simulink model "UZ_EnDat_be4_adding_bidirectional_clk_shift"  (R2024a)
settings: Solver=FixedStepDiscrete  StartTime=0  StopTime=0.02  FixedStep=1.0E-8  RelTol=1e-3
model workspace (MAT data in the model file):
  Select = 0
libraries: hdlsllib x776, simulink x28, simulink_extras x3
(part 2 of 9)

== system UZ_EnDat_be4_adding_bidirectional_clk_shift/UZ_ENDAT/CRC_Check ==
  set : Inport
  data : Inport  Port=2  OutDataTypeStr=boolean
  clk : Inport  Port=3  OutDataTypeStr=boolean
  Constant : Constant  OutDataTypeStr=boolean  SampleTime=-1
  Constant1 : Constant  Value=0  OutDataTypeStr=boolean  SampleTime=-1
  DFF1 : Subsystem
  DFF2 : Subsystem
  DFF3 : Subsystem
  DFF4 : Subsystem
  DFF5 : Subsystem
  Logical Operator : Logic  Operator=OR  AllPortsSameDT=off  OutDataTypeStr=boolean
  Logical Operator{1..2,5..6} (4 alike) : Logic  AllPortsSameDT=off  OutDataTypeStr=boolean
  Logical Operator3 : Logic  Operator=NOT  AllPortsSameDT=off  OutDataTypeStr=boolean
  Logical Operator4 : Logic  Operator=NOT  AllPortsSameDT=off  OutDataTypeStr=boolean
  Memory : Memory  InheritSampleTime=on
  Memory1 : Memory  InheritSampleTime=on
  Relational Operator : RelationalOperator  Operator===  OutDataTypeStr=boolean  InputSameDT=off
  Relational Operator1 : RelationalOperator  Operator===  OutDataTypeStr=boolean  InputSameDT=off
  Relational Operator2 : RelationalOperator  Operator===  OutDataTypeStr=boolean  InputSameDT=off
  Terminator{,1..3} (4 alike) : Terminator
  crc : Outport
  CRC1 : Outport  Port=2
  CRC2 : Outport  Port=3
  CRC3 : Outport  Port=4
  CRC4 : Outport  Port=5
  CRC5 : Outport  Port=6
  wires:
  Logical Operator/1 -> crc/1
  Logical Operator2/1 -> Logical Operator/2
  Logical Operator1/1 -> Logical Operator/1
  data/1 -> Relational Operator/2, Logical Operator1/1
  Logical Operator3/1 -> Logical Operator1/2
  Logical Operator4/1 -> Logical Operator3/1, Logical Operator2/2
  Logical Operator5/1 -> Memory1/1
  Relational Operator/1 -> DFF1/3(D), Logical Operator6/1
  clk/1 -> DFF1/2(CLK), DFF2/2(CLK), DFF3/2(CLK), DFF5/2(CLK), DFF4/2(CLK)
  set/1 -> Logical Operator6/2, Logical Operator5/2, Logical Operator4/1
  DFF1/1(OQ) -> Relational Operator1/1, CRC1/1
  Logical Operator6/1 -> Memory/1
  Relational Operator1/1 -> DFF2/3(D)
  Relational Operator2/1 -> DFF4/3(D)
  DFF3/1(OQ) -> CRC3/1, Relational Operator2/1
  DFF4/1(OQ) -> DFF5/3(D), CRC4/1
  DFF5/2(NOQ) -> Logical Operator2/1
  DFF5/1(OQ) -> Logical Operator5/1, CRC5/1
  DFF2/1(OQ) -> DFF3/3(D), CRC2/1
  DFF1/2(NOQ) -> Terminator/1
  DFF2/2(NOQ) -> Terminator1/1
  DFF3/2(NOQ) -> Terminator2/1
  DFF4/2(NOQ) -> Terminator3/1
  Constant/1 -> DFF3/1(SET), DFF5/1(SET), DFF4/1(SET), DFF2/1(SET), DFF1/1(SET)
  Constant1/1 -> DFF5/4(RST), DFF4/4(RST), DFF3/4(RST), DFF2/4(RST), DFF1/4(RST)
  Memory/1 -> Relational Operator2/2, Relational Operator1/2
  Memory1/1 -> Relational Operator/1

== system UZ_EnDat_be4_adding_bidirectional_clk_shift/UZ_ENDAT/DATA2CLOCKSYNCER ==
  In1 : Inport
  FAKTOR : Inport  Port=2
  Constant : Constant  Value=100  OutDataTypeStr=uint16  SampleTime=-1
  Constant1 : Constant  Value=45  OutDataTypeStr=uint16  SampleTime=-1
  Constant2 : Constant  Value=2  OutDataTypeStr=uint16  SampleTime=-1
  Constant23 : Constant  Value=20  OutDataTypeStr=uint16  SampleTime=-1
  Constant24 : Constant  Value=29  OutDataTypeStr=uint16  SampleTime=-1
  Constant3 : Constant  Value=12  OutDataTypeStr=uint16  SampleTime=-1
  Constant4 : Constant  Value=4  OutDataTypeStr=uint16  SampleTime=-1
  Constant7 : Constant  Value=8  OutDataTypeStr=uint16  SampleTime=-1
  Display15 : Display
  Divide : Product  Inputs=*/  OutDataTypeStr=uint16  RndMeth=Simplest  SaturateOnIntegerOverflow=on
  Multiport Switch1 : MultiPortSwitch  DataPortOrder=Zero-based contiguous  Inputs=7  DataPortIndices={8,16,32,64}  zeroidx=on  SaturateOnIntegerOverflow=off  InputSameDT=off
  Product : Product  RndMeth=Simplest  SaturateOnIntegerOverflow=on  OutDataTypeStr=Inherit: Same as first input
  Out1 : Outport
  wires:
  In1/1 -> Multiport Switch1/1
  FAKTOR/1 -> Product/2
  Constant/1 -> Divide/2
  Multiport Switch1/1 -> Product/1
  Product/1 -> Divide/1
  Constant2/1 -> Multiport Switch1/2
  Constant4/1 -> Multiport Switch1/3
  Constant7/1 -> Multiport Switch1/4
  Constant3/1 -> Multiport Switch1/5
  Constant23/1 -> Multiport Switch1/6
  Constant24/1 -> Multiport Switch1/7
  Constant1/1 -> Multiport Switch1/8
  Divide/1 -> Display15/1, Out1/1

== system UZ_EnDat_be4_adding_bidirectional_clk_shift/UZ_ENDAT/DATAFLOWCHGER ==
  CLKSEL : Inport
  FACTOR : Inport  Port=2
  Constant : Constant  Value=100  OutDataTypeStr=uint16  SampleTime=-1
  Constant{14..18,27..28} (7 alike) : Constant  Value=10  OutDataTypeStr=uint16  SampleTime=-1
  Divide : Product  Inputs=*/  InputSameDT=on  OutDataTypeStr=uint16  RndMeth=Simplest  SaturateOnIntegerOverflow=on
  Multiport Switch2 : MultiPortSwitch  DataPortOrder=Zero-based contiguous  Inputs=7  DataPortIndices={8,16,32,64}  zeroidx=on  SaturateOnIntegerOverflow=off  InputSameDT=off
  Product : Product  RndMeth=Simplest  SaturateOnIntegerOverflow=on  OutDataTypeStr=Inherit: Same as first input
  Output : Outport
  wires:
  Product/1 -> Divide/1
  CLKSEL/1 -> Multiport Switch2/1
  FACTOR/1 -> Product/2
  Constant/1 -> Divide/2
  Divide/1 -> Output/1
  Multiport Switch2/1 -> Product/1
  Constant15/1 -> Multiport Switch2/2
  Constant16/1 -> Multiport Switch2/3
  Constant17/1 -> Multiport Switch2/4
  Constant18/1 -> Multiport Switch2/5
  Constant27/1 -> Multiport Switch2/6
  Constant28/1 -> Multiport Switch2/7
  Constant14/1 -> Multiport Switch2/8

== system UZ_EnDat_be4_adding_bidirectional_clk_shift/UZ_ENDAT/DIFFBUILDER ==
  DATAT0 : Inport
  DATAT1 : Inport  Port=2
  DATAT2 : Inport  Port=3
  Trigger : TriggerPort  VariantControl=(inherit)  OutputDataType=int8  InitialTriggerSignalState=positive
  Subtract : Sum  Inputs=+-  OutDataTypeStr=int32  InputSameDT=on  RndMeth=Simplest
  Subtract1 : Sum  Inputs=+-  OutDataTypeStr=int32  InputSameDT=on  RndMeth=Simplest
  DIFT1T0 : Outport  InitialOutput=0
  DIFT2T0 : Outport  Port=2  InitialOutput=0
  wires:
  DATAT1/1 -> Subtract/2
  DATAT0/1 -> Subtract/1, Subtract1/1
  Subtract/1 -> DIFT1T0/1
  Subtract1/1 -> DIFT2T0/1
  DATAT2/1 -> Subtract1/2

== system UZ_EnDat_be4_adding_bidirectional_clk_shift/UZ_ENDAT/INITIALOFF ==
  CLKAUX : Inport
  CLK : Inport  Port=2
  DATAWR : Inport  Port=3
  DATA : Inport  Port=4
  CLKWR : Inport  Port=5
  FACTOR : Inport  Port=6
  Constant : Constant  Value=0  OutDataTypeStr=boolean  SampleTime=-1
  Display : Display
  Memory : Memory  InheritSampleTime=on
  Multiport Switch{,1..3} (4 alike) : MultiPortSwitch  DataPortOrder=Zero-based contiguous  Inputs=2  zeroidx=on  SaturateOnIntegerOverflow=off  InputSameDT=off
  Relational Operator : RelationalOperator  Operator=<  OutDataTypeStr=boolean  InputSameDT=off
  Subsystem : Subsystem
  Subsystem6 : Subsystem
  CLK_OUT : Outport
  DATAWR_OUT : Outport  Port=2
  DATA_OUT : Outport  Port=3
  CLKWR_OUT : Outport  Port=4
  wires:
  Relational Operator/1 -> Multiport Switch3/1, Multiport Switch2/1, Multiport Switch1/1, Multiport Switch/1, Memory/1
  CLK/1 -> Multiport Switch/2
  Multiport Switch/1 -> CLK_OUT/1
  CLKAUX/1 -> Subsystem/Trigger
  Constant/1 -> Multiport Switch3/3, Multiport Switch2/3, Multiport Switch1/3, Multiport Switch/3
  Multiport Switch1/1 -> DATAWR_OUT/1
  Multiport Switch2/1 -> DATA_OUT/1
  Multiport Switch3/1 -> CLKWR_OUT/1
  DATAWR/1 -> Multiport Switch1/2
  DATA/1 -> Multiport Switch2/2
  CLKWR/1 -> Multiport Switch3/2
  Subsystem6/1(out) -> Relational Operator/2
  FACTOR/1 -> Subsystem6/1(FACTOR)
  Subsystem/1(count) -> Display/1, Relational Operator/1
  Memory/1 -> Subsystem/1(In1)

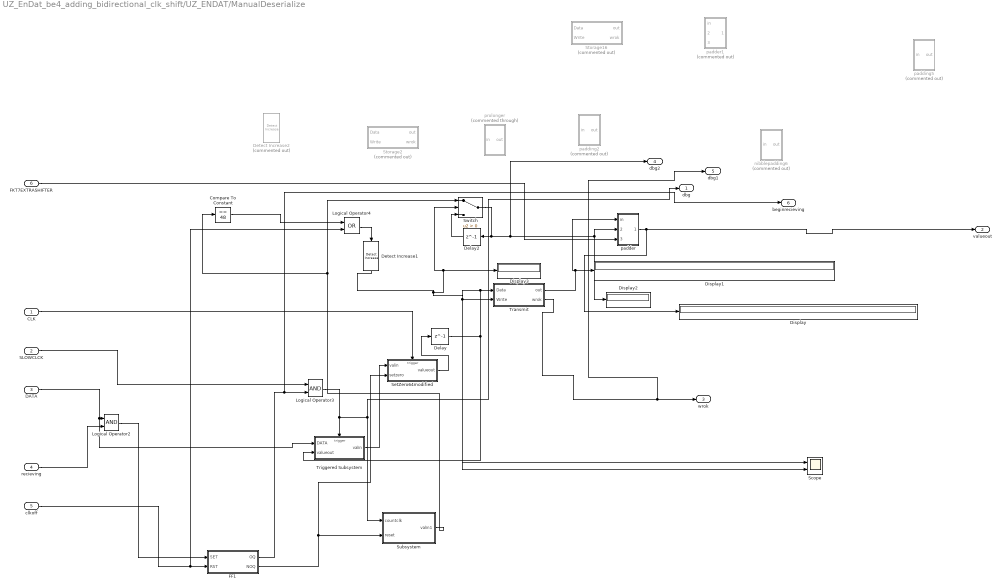
== system UZ_EnDat_be4_adding_bidirectional_clk_shift/UZ_ENDAT/ManualDeserialize ==
  CLK : Inport
  SLOWCLCK : Inport  Port=2
  DATA : Inport  Port=3
  recieving : Inport  Port=4  OutMin=0  OutMax=1  OutDataTypeStr=boolean
  clkoff : Inport  Port=5  OutMin=0  OutMax=1  OutDataTypeStr=boolean
  FKT7EXTRASHIFTER : Inport  Port=6
  Compare To Constant : hdlsllib/Logic and Bit Operations/Compare To Constant  relop===  const=48  OutDataTypeStr=boolean
  Delay : Delay  DelayLength=1
  Delay2 : Delay  DelayLength=1
  Detect Increase1 : simulink/Logic and Bit Operations/Detect Increase  vinit=0  OutDataTypeStr=boolean
      settings: LibrarySourceBlock=|
      | hdlsllib/Logic and Bit
      | Operations/Detect
      | Increase
  Detect Increase2 : simulink/Logic and Bit Operations/Detect Increase  Commented=on  vinit=0.0  InputProcessing=Columns as channels (frame based)  OutDataTypeStr=boolean
      settings: LibrarySourceBlock=|
      | hdlsllib/Logic and Bit
      | Operations/Detect
      | Increase
  Display{,1..3} (4 alike) : Display
      Display settings: Format=binary (Stored Integer)
      Display1 settings: Format=binary (Stored Integer)
  FF1 : Subsystem  TreatAsAtomicUnit=on
      settings: LibrarySourceBlock=|
      | hdlsllib/Ports &
      | Subsystems/Triggered
      | Subsystem
  Logical Operator2 : Logic  AllPortsSameDT=off  OutDataTypeStr=boolean
  Logical Operator3 : Logic  AllPortsSameDT=off  OutDataTypeStr=boolean
  Logical Operator4 : Logic  Operator=OR  AllPortsSameDT=off  OutDataTypeStr=boolean
  Scope : Scope  NumInputPorts=2
  SetZero64modified : Subsystem
  Storage16 : Subsystem  Commented=on
      settings: LibrarySourceBlock=|
      | hdlsllib/Ports &
      | Subsystems/Subsystem
  Storage2 : Subsystem  Commented=on
      settings: LibrarySourceBlock=|
      | hdlsllib/Ports &
      | Subsystems/Subsystem
  Subsystem : Subsystem
  Switch : Switch  Criteria=u2 > Threshold  SaturateOnIntegerOverflow=off  InputSameDT=off
  Transmit : Subsystem
      settings: LibrarySourceBlock=|
      | hdlsllib/Ports &
      | Subsystems/Subsystem
  Triggered Subsystem : Subsystem  TreatAsAtomicUnit=on
      settings: LibrarySourceBlock=|
      | hdlsllib/Ports &
      | Subsystems/Triggered
      | Subsystem
  nibblepadding6 : Subsystem  Commented=on
  padder : Subsystem
  padder1 : Subsystem  Commented=on
  padding2 : Subsystem  Commented=on
  padding5 : Subsystem  Commented=on
  prolonger : Subsystem  Commented=through
  dbg : Outport  OutDataTypeStr=boolean  VectorParamsAs1DForOutWhenUnconnected=off
  valueout : Outport  Port=2  OutDataTypeStr=uint64
  wrok : Outport  Port=3  OutDataTypeStr=boolean
  dbg2 : Outport  Port=4  OutDataTypeStr=uint8  VectorParamsAs1DForOutWhenUnconnected=off
  dbg1 : Outport  Port=5  OutDataTypeStr=boolean  VectorParamsAs1DForOutWhenUnconnected=off
  beginrecieving : Outport  Port=6  OutDataTypeStr=boolean  VectorParamsAs1DForOutWhenUnconnected=off
  wires:
  SetZero64modified/1(valueout) -> Delay/1
  CLK/1 -> SetZero64modified/Trigger
  SLOWCLCK/1 -> Logical Operator3/1
  Triggered Subsystem/1(valin) -> SetZero64modified/1(valin)
  Logical Operator3/1 -> dbg/1, Subsystem/1(countclk), Triggered Subsystem/Trigger
  Logical Operator2/1 -> FF1/1(SET)
  FF1/1(OQ) -> beginrecieving/1, Logical Operator3/2
  recieving/1 -> Logical Operator2/2
  FF1/2(NOQ) -> Subsystem/2(reset), SetZero64modified/2(setzero)
  Compare To Constant/1 -> Logical Operator4/1
  Delay2/1 -> Switch/3
  clkoff/1 -> Logical Operator4/2, FF1/2(RST)
  DATA/1 -> Triggered Subsystem/1(DATA), Logical Operator2/1
  Delay/1 -> Transmit/1(Data), Scope/2, Triggered Subsystem/2(valueout)
  Transmit/1(out) -> padder/1(in), Display1/1
  padder/1(out) -> valueout/1, Display/1
  Switch/1 -> Delay2/1, dbg2/1, padder/2(CTR), Display2/1
  Transmit/2(wrok) -> dbg1/1, wrok/1
  FKT7EXTRASHIFTER/1 -> padder/3(in1)
  Logical Operator4/1 -> Detect Increase1/1
  Subsystem/1(valin1) -> Switch/1, Compare To Constant/1
  Detect Increase1/1 -> Transmit/2(Write), Scope/1, Switch/2, Display3/1

== system UZ_EnDat_be4_adding_bidirectional_clk_shift/UZ_ENDAT/ManualSerializeWrap ==
  CLK : Inport
  SLOWCLCK : Inport  Port=2
  DATA : Inport  Port=3
  reset : Inport  Port=4
  Enable : EnablePort
  ManualSerializer : Subsystem
      settings: LibrarySourceBlock=|
      | hdlsllib/Ports &
      | Subsystems/Subsystem
  valin : Outport  InitialOutput=0
  wires:
  CLK/1 -> ManualSerializer/1(CLK)
  DATA/1 -> ManualSerializer/3(DATA)
  reset/1 -> ManualSerializer/4(reset)
  SLOWCLCK/1 -> ManualSerializer/2(SLOWCLCK)
  ManualSerializer/1(valin) -> valin/1

== system UZ_EnDat_be4_adding_bidirectional_clk_shift/UZ_ENDAT/OUTPUTCONTROLCONTINIOUS ==
  CLKCNT : Inport
  CLKS2DATAFLOWCHG : Inport  Port=2
  CLK2ENDOFTRANSMISSION : Inport  Port=3
  OPENCOM : Inport  Port=4
  CLKCNTNOSTOP : Inport  Port=5
  RECOVERYTIME : Inport  Port=6  OutDataTypeStr=uint16
  Add : Sum  OutDataTypeStr=uint16  AccumDataTypeStr=uint16
  Constant : Constant  Value=0  OutDataTypeStr=uint8  SampleTime=-1
  Logical Operator : Logic  Operator=OR  AllPortsSameDT=off  OutDataTypeStr=boolean
  Logical Operator1 : Logic  AllPortsSameDT=off  OutDataTypeStr=boolean
  Logical Operator6 : Logic  Operator=NOT  Inputs=3  AllPortsSameDT=off  OutDataTypeStr=boolean
  Relational Operator : RelationalOperator  Operator=<=  OutDataTypeStr=boolean  RndMeth=Simplest  InputSameDT=off
  Relational Operator1 : RelationalOperator  OutDataTypeStr=boolean  RndMeth=Simplest  InputSameDT=off
  Relational Operator2 : RelationalOperator  OutDataTypeStr=boolean  RndMeth=Simplest  InputSameDT=off
  Relational Operator3 : RelationalOperator  OutDataTypeStr=boolean  RndMeth=Simplest  InputSameDT=off
  CLKOFF : Outport  OutDataTypeStr=boolean
  DATAINV : Outport  Port=2  OutDataTypeStr=boolean
  RESETCNT : Outport  Port=3  OutDataTypeStr=boolean
  wires:
  CLKCNT/1 -> Relational Operator1/1, Relational Operator2/1, Relational Operator/1
  CLKS2DATAFLOWCHG/1 -> Relational Operator/2
  Relational Operator/1 -> Logical Operator1/1
  CLK2ENDOFTRANSMISSION/1 -> Add/1, Relational Operator1/2
  Relational Operator1/1 -> Logical Operator/2
  Logical Operator/1 -> CLKOFF/1
  OPENCOM/1 -> Logical Operator6/1
  Logical Operator6/1 -> Logical Operator/1
  Relational Operator2/1 -> Logical Operator1/2
  Constant/1 -> Relational Operator2/2
  Logical Operator1/1 -> DATAINV/1
  RECOVERYTIME/1 -> Add/2
  Add/1 -> Relational Operator3/2
  Relational Operator3/1 -> RESETCNT/1
  CLKCNTNOSTOP/1 -> Relational Operator3/1

== system UZ_EnDat_be4_adding_bidirectional_clk_shift/UZ_ENDAT/RECOVERYTIMESELECTOR ==
  note: 200khz = 6
      | 1,5mhz = 12
      | 3 mhz = 8
  In1 : Inport
  FAKTOR : Inport  Port=2
  Constant : Constant  Value=100  OutDataTypeStr=uint16  SampleTime=-1
  Constant19 : Constant  Value=96  OutDataTypeStr=uint16  SampleTime=-1
  Constant20 : Constant  Value=48  OutDataTypeStr=uint16  SampleTime=-1
  Constant21 : Constant  Value=192  OutDataTypeStr=uint16  SampleTime=-1
  Constant22 : Constant  Value=255  OutDataTypeStr=uint16  SampleTime=-1
  Constant25 : Constant  Value=24  OutDataTypeStr=uint16  SampleTime=-1
  Constant26 : Constant  Value=12  OutDataTypeStr=uint16  SampleTime=-1
  Constant5 : Constant  Value=6  OutDataTypeStr=uint16  SampleTime=-1
  Divide : Product  Inputs=*/  InputSameDT=on  OutDataTypeStr=uint16  RndMeth=Simplest  SaturateOnIntegerOverflow=on
  Multiport Switch3 : MultiPortSwitch  DataPortOrder=Zero-based contiguous  Inputs=7  DataPortIndices={8,16,32,64}  zeroidx=on  SaturateOnIntegerOverflow=off  InputSameDT=off
  Product : Product  RndMeth=Simplest  SaturateOnIntegerOverflow=on  OutDataTypeStr=Inherit: Same as first input
  Out1 : Outport
  wires:
  In1/1 -> Multiport Switch3/1
  Constant5/1 -> Multiport Switch3/8
  FAKTOR/1 -> Product/2
  Constant/1 -> Divide/2
  Divide/1 -> Out1/1
  Multiport Switch3/1 -> Product/1
  Product/1 -> Divide/1
  Constant26/1 -> Multiport Switch3/7
  Constant25/1 -> Multiport Switch3/6
  Constant20/1 -> Multiport Switch3/5
  Constant19/1 -> Multiport Switch3/4
  Constant21/1 -> Multiport Switch3/3
  Constant22/1 -> Multiport Switch3/2

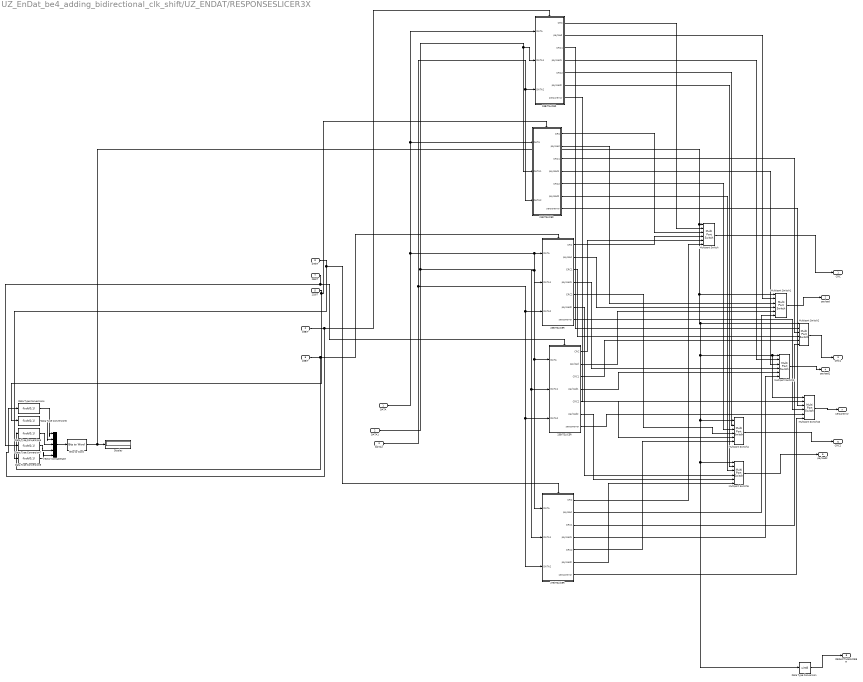
== system UZ_EnDat_be4_adding_bidirectional_clk_shift/UZ_ENDAT/RESPONSESLICER3X ==
  DATA : Inport
  DATA1 : Inport  Port=2
  DATA2 : Inport  Port=3
  19BIT : Inport  Port=4  OutDataTypeStr=boolean
  21BIT : Inport  Port=5  OutDataTypeStr=boolean
  23BIT : Inport  Port=6  OutDataTypeStr=boolean
  25BIT : Inport  Port=7  OutDataTypeStr=boolean
  27BIT : Inport  Port=8  OutDataTypeStr=boolean
  19BITSLICER : Subsystem
  21BITSLICER : Subsystem
  23BITSLICER : Subsystem
  25BITSLICER : Subsystem
  27BITSLICER : Subsystem
  Bits to Word : hdlsllib/Logic and Bit Operations/Bits to Word
  Data Type Conversion : DataTypeConversion  OutDataTypeStr=uint8  RndMeth=Nearest  SaturateOnIntegerOverflow=off
  Data Type Conversion{4..8} (5 alike) : DataTypeConversion  OutMax=1  OutDataTypeStr=fixdt(0,1)  SaturateOnIntegerOverflow=off  RndMeth=Floor
  Display : Display
  Multiport Switch{,1..5,10} (7 alike) : MultiPortSwitch  DataPortOrder=Specify indices  Inputs=5  DataPortIndices={1,2,4,8,16}  DiagnosticForDefault=Warning  RndMeth=Simplest  SaturateOnIntegerOverflow=off  InputSameDT=off
  Vector Concatenate : Concatenate  NumInputs=5
  CRC : Outport
  payload : Outport  Port=2
  CRC1 : Outport  Port=3
  payload1 : Outport  Port=4
  CRC2 : Outport  Port=5
  payload2 : Outport  Port=6
  sensorerror : Outport  Port=7  OutDataTypeStr=boolean
  DBGACTIVENUMBER : Outport  Port=8
  wires:
  23BITSLICER/1(CRC) -> Multiport Switch/4
  DATA1/1 -> 19BITSLICER/2(DATA1), 21BITSLICER/2(DATA1), 23BITSLICER/2(DATA1), 27BITSLICER/2(DATA1), 25BITSLICER/2(DATA1)
  DATA2/1 -> 21BITSLICER/3(DATA2), 19BITSLICER/3(DATA2), 23BITSLICER/3(DATA2), 27BITSLICER/3(DATA2), 25BITSLICER/3(DATA2)
  DATA/1 -> 19BITSLICER/1(DATA), 21BITSLICER/1(DATA), 23BITSLICER/1(DATA), 27BITSLICER/1(DATA), 25BITSLICER/1(DATA)
  Multiport Switch2/1 -> CRC1/1
  Multiport Switch3/1 -> payload1/1
  Multiport Switch4/1 -> CRC2/1
  Multiport Switch5/1 -> payload2/1
  Multiport Switch1/1 -> payload/1
  Multiport Switch/1 -> CRC/1
  19BIT/1 -> 19BITSLICER/Enable, Data Type Conversion4/1
  Data Type Conversion6/1 -> Vector Concatenate/3
  25BIT/1 -> Data Type Conversion7/1, 25BITSLICER/Enable
  Vector Concatenate/1 -> Bits to Word/1
  23BIT/1 -> 23BITSLICER/Enable, Data Type Conversion6/1
  Data Type Conversion4/1 -> Vector Concatenate/1
  Data Type Conversion7/1 -> Vector Concatenate/4
  27BIT/1 -> 27BITSLICER/Enable, Data Type Conversion8/1
  Data Type Conversion5/1 -> Vector Concatenate/2
  21BIT/1 -> 21BITSLICER/Enable, Data Type Conversion5/1
  Data Type Conversion8/1 -> Vector Concatenate/5
  19BITSLICER/1(CRC) -> Multiport Switch/2
  21BITSLICER/1(CRC) -> Multiport Switch/3
  25BITSLICER/1(CRC) -> Multiport Switch/5
  27BITSLICER/1(CRC) -> Multiport Switch/6
  23BITSLICER/2(payload) -> Multiport Switch1/4
  19BITSLICER/2(payload) -> Multiport Switch1/2
  21BITSLICER/2(payload) -> Multiport Switch1/3
  25BITSLICER/2(payload) -> Multiport Switch1/5
  27BITSLICER/2(payload) -> Multiport Switch1/6
  23BITSLICER/3(CRC1) -> Multiport Switch2/4
  21BITSLICER/3(CRC1) -> Multiport Switch2/3
  19BITSLICER/3(CRC1) -> Multiport Switch2/2
  25BITSLICER/3(CRC1) -> Multiport Switch2/5
  27BITSLICER/3(CRC1) -> Multiport Switch2/6
  23BITSLICER/4(payload1) -> Multiport Switch3/4
  21BITSLICER/4(payload1) -> Multiport Switch3/3
  19BITSLICER/4(payload1) -> Multiport Switch3/2
  25BITSLICER/4(payload1) -> Multiport Switch3/5
  27BITSLICER/4(payload1) -> Multiport Switch3/6
  23BITSLICER/5(CRC2) -> Multiport Switch4/4
  19BITSLICER/5(CRC2) -> Multiport Switch4/2
  21BITSLICER/5(CRC2) -> Multiport Switch4/3
  25BITSLICER/5(CRC2) -> Multiport Switch4/5
  27BITSLICER/5(CRC2) -> Multiport Switch4/6
  23BITSLICER/6(payload2) -> Multiport Switch5/4
  19BITSLICER/6(payload2) -> Multiport Switch5/2
  21BITSLICER/6(payload2) -> Multiport Switch5/3
  25BITSLICER/6(payload2) -> Multiport Switch5/5
  27BITSLICER/6(payload2) -> Multiport Switch5/6
  Multiport Switch10/1 -> sensorerror/1
  25BITSLICER/7(sensorerror) -> Multiport Switch10/5
  27BITSLICER/7(sensorerror) -> Multiport Switch10/6
  23BITSLICER/7(sensorerror) -> Multiport Switch10/4
  21BITSLICER/7(sensorerror) -> Multiport Switch10/3
  19BITSLICER/7(sensorerror) -> Multiport Switch10/2
  Data Type Conversion/1 -> DBGACTIVENUMBER/1
  Bits to Word/1 -> Data Type Conversion/1, Multiport Switch5/1, Multiport Switch4/1, Multiport Switch10/1, Multiport Switch3/1, Multiport Switch2/1, Multiport Switch1/1, Multiport Switch/1, Display/1

== system UZ_EnDat_be4_adding_bidirectional_clk_shift/UZ_ENDAT/SetZeroBool ==
  valin : Inport
  setzero : Inport  Port=2  OutDataTypeStr=boolean
  Trigger : TriggerPort  TriggerType=either  VariantControl=(inherit)
  Constant1 : Constant  OutDataTypeStr=boolean  SampleTime=-1
  Constant2 : Constant  Value=0  OutDataTypeStr=boolean  SampleTime=-1
  Index Vector1 : MultiPortSwitch  DataPortOrder=Zero-based contiguous  Inputs=2  zeroidx=on  SaturateOnIntegerOverflow=off  InputSameDT=off
  Logical Operator : Logic  AllPortsSameDT=off  OutDataTypeStr=boolean
  valueout : Outport  InitialOutput=1  VectorParamsAs1DForOutWhenUnconnected=off
  wires:
  Index Vector1/1 -> Logical Operator/1
  valin/1 -> Logical Operator/2
  Logical Operator/1 -> valueout/1
  Constant1/1 -> Index Vector1/2
  Constant2/1 -> Index Vector1/3
  setzero/1 -> Index Vector1/1

== system UZ_EnDat_be4_adding_bidirectional_clk_shift/UZ_ENDAT/SetZeroBool1 ==
  valin : Inport
  setzero : Inport  Port=2  OutDataTypeStr=boolean
  Trigger : TriggerPort  TriggerType=either  VariantControl=(inherit)
  Constant1 : Constant  OutDataTypeStr=boolean  SampleTime=-1
  Constant2 : Constant  Value=0  OutDataTypeStr=boolean  SampleTime=-1
  Index Vector1 : MultiPortSwitch  DataPortOrder=Zero-based contiguous  Inputs=2  zeroidx=on  SaturateOnIntegerOverflow=off  InputSameDT=off
  Logical Operator : Logic  AllPortsSameDT=off  OutDataTypeStr=boolean
  valueout : Outport  InitialOutput=1  VectorParamsAs1DForOutWhenUnconnected=off
  wires:
  Index Vector1/1 -> Logical Operator/1
  valin/1 -> Logical Operator/2
  Logical Operator/1 -> valueout/1
  Constant1/1 -> Index Vector1/2
  Constant2/1 -> Index Vector1/3
  setzero/1 -> Index Vector1/1

== system UZ_EnDat_be4_adding_bidirectional_clk_shift/UZ_ENDAT/SetZeroBool2 ==
  valin : Inport
  setzero : Inport  Port=2  OutDataTypeStr=boolean
  Trigger : TriggerPort  TriggerType=either  VariantControl=(inherit)
  Constant1 : Constant  OutDataTypeStr=boolean  SampleTime=-1
  Constant2 : Constant  Value=0  OutDataTypeStr=boolean  SampleTime=-1
  Index Vector1 : MultiPortSwitch  DataPortOrder=Zero-based contiguous  Inputs=2  zeroidx=on  SaturateOnIntegerOverflow=off  InputSameDT=off
  Logical Operator : Logic  AllPortsSameDT=off  OutDataTypeStr=boolean
  valueout : Outport  InitialOutput=1  VectorParamsAs1DForOutWhenUnconnected=off
  wires:
  Index Vector1/1 -> Logical Operator/1
  valin/1 -> Logical Operator/2
  Logical Operator/1 -> valueout/1
  Constant1/1 -> Index Vector1/2
  Constant2/1 -> Index Vector1/3
  setzero/1 -> Index Vector1/1

== system UZ_EnDat_be4_adding_bidirectional_clk_shift/UZ_ENDAT/SetZeroBool3 ==
  valin : Inport
  setzero : Inport  Port=2  OutDataTypeStr=boolean
  Trigger : TriggerPort  TriggerType=either  VariantControl=(inherit)
  Constant1 : Constant  OutDataTypeStr=boolean  SampleTime=-1
  Constant2 : Constant  Value=0  OutDataTypeStr=boolean  SampleTime=-1
  Index Vector1 : MultiPortSwitch  DataPortOrder=Zero-based contiguous  Inputs=2  zeroidx=on  SaturateOnIntegerOverflow=off  InputSameDT=off
  Logical Operator : Logic  AllPortsSameDT=off  OutDataTypeStr=boolean
  valueout : Outport  InitialOutput=1  VectorParamsAs1DForOutWhenUnconnected=off
  wires:
  Index Vector1/1 -> Logical Operator/1
  valin/1 -> Logical Operator/2
  Logical Operator/1 -> valueout/1
  Constant1/1 -> Index Vector1/2
  Constant2/1 -> Index Vector1/3
  setzero/1 -> Index Vector1/1

== system UZ_EnDat_be4_adding_bidirectional_clk_shift/UZ_ENDAT/SetZeroBool4 ==
  valin : Inport
  setzero : Inport  Port=2  OutDataTypeStr=boolean
  Trigger : TriggerPort  TriggerType=either  VariantControl=(inherit)
  Constant1 : Constant  OutDataTypeStr=boolean  SampleTime=-1
  Constant2 : Constant  Value=0  OutDataTypeStr=boolean  SampleTime=-1
  Index Vector1 : MultiPortSwitch  DataPortOrder=Zero-based contiguous  Inputs=2  zeroidx=on  SaturateOnIntegerOverflow=off  InputSameDT=off
  Logical Operator : Logic  AllPortsSameDT=off  OutDataTypeStr=boolean
  valueout : Outport  InitialOutput=1  VectorParamsAs1DForOutWhenUnconnected=off
  wires:
  Index Vector1/1 -> Logical Operator/1
  valin/1 -> Logical Operator/2
  Logical Operator/1 -> valueout/1
  Constant1/1 -> Index Vector1/2
  Constant2/1 -> Index Vector1/3
  setzero/1 -> Index Vector1/1

== system UZ_EnDat_be4_adding_bidirectional_clk_shift/UZ_ENDAT/SetZeroBool5 ==
  valin : Inport
  setzero : Inport  Port=2  OutDataTypeStr=boolean
  Trigger : TriggerPort  TriggerType=either  VariantControl=(inherit)
  Constant1 : Constant  OutDataTypeStr=boolean  SampleTime=-1
  Constant2 : Constant  Value=0  OutDataTypeStr=boolean  SampleTime=-1
  Index Vector1 : MultiPortSwitch  DataPortOrder=Zero-based contiguous  Inputs=2  zeroidx=on  SaturateOnIntegerOverflow=off  InputSameDT=off
  Logical Operator : Logic  AllPortsSameDT=off  OutDataTypeStr=boolean
  valueout : Outport  InitialOutput=1  VectorParamsAs1DForOutWhenUnconnected=off
  wires:
  Index Vector1/1 -> Logical Operator/1
  valin/1 -> Logical Operator/2
  Logical Operator/1 -> valueout/1
  Constant1/1 -> Index Vector1/2
  Constant2/1 -> Index Vector1/3
  setzero/1 -> Index Vector1/1

== system UZ_EnDat_be4_adding_bidirectional_clk_shift/UZ_ENDAT/Storage16 ==
  Data : Inport
  Write : Inport  Port=2  OutDataTypeStr=boolean
  Compare To Zero : hdlsllib/Logic and Bit Operations/Compare To Zero  relop===  OutDataTypeStr=boolean
  Logical Operator : Logic  Operator=NOT  AllPortsSameDT=off  OutDataTypeStr=boolean
  Logical Operator1 : Logic  Inputs=3  AllPortsSameDT=off  OutDataTypeStr=boolean
  Logical Operator2 : Logic  Operator=NOT  AllPortsSameDT=off  OutDataTypeStr=boolean
  Logical Operator3 : Logic  AllPortsSameDT=off  OutDataTypeStr=boolean
  Relational Operator : RelationalOperator  Operator===  OutDataTypeStr=boolean  InputSameDT=off
  Single Port RAM System : hdlsllib/HDL RAMs/Single Port RAM System  RAMType=Single port  AsyncRead=off  WriteOutputValue=Old data  RAMInitialValue=0  allowBusInputs=off  WritesHaveOutput=on  NumReads=0  NumWrites=1  SimulateUsing=Code generation
  adress : Constant  Value=5  OutDataTypeStr=uint8  SampleTime=-1
  out : Outport
  wrok : Outport  Port=2  OutDataTypeStr=boolean
  wires:
  Single Port RAM System/1 -> Relational Operator/1, out/1
  Data/1 -> Compare To Zero/1, Single Port RAM System/1, Relational Operator/2
  adress/1 -> Single Port RAM System/2
  Relational Operator/1 -> Logical Operator3/1, Logical Operator/1
  Logical Operator/1 -> Logical Operator1/2
  Write/1 -> Logical Operator1/1
  Compare To Zero/1 -> Logical Operator2/1
  Logical Operator2/1 -> Logical Operator3/2, Logical Operator1/3
  Logical Operator1/1 -> Single Port RAM System/3
  Logical Operator3/1 -> wrok/1

== system UZ_EnDat_be4_adding_bidirectional_clk_shift/UZ_ENDAT/Subsystem1 ==
  in : Inport
  Enable : EnablePort
  Bits to Word1 : hdlsllib/Logic and Bit Operations/Bits to Word
  out : Outport  InitialOutput=0
  wires:
  Bits to Word1/1 -> out/1
  in/1 -> Bits to Word1/1

== system UZ_EnDat_be4_adding_bidirectional_clk_shift/UZ_ENDAT/Subsystem6 ==
  In1 : Inport  OutDataTypeStr=uint16
  FACTOR : Inport  Port=2  OutMin=0  OutMax=60000
  Constant : Constant  Value=100  OutDataTypeStr=uint16  SampleTime=-1
  Divide : Product  Inputs=*/  OutDataTypeStr=uint16  RndMeth=Simplest  SaturateOnIntegerOverflow=on
  Product : Product  OutDataTypeStr=uint16  RndMeth=Simplest  SaturateOnIntegerOverflow=on
  Out1 : Outport
  wires:
  In1/1 -> Product/1
  FACTOR/1 -> Product/2
  Constant/1 -> Divide/2
  Product/1 -> Divide/1
  Divide/1 -> Out1/1

== system UZ_EnDat_be4_adding_bidirectional_clk_shift/UZ_ENDAT/ageprovider ==
  wrok : Inport  OutDataTypeStr=boolean
  recieving : Inport  Port=2  OutDataTypeStr=boolean
  altmode : Inport  Port=3  OutDataTypeStr=boolean
  Constant : Constant  Value=10  OutDataTypeStr=uint8  SampleTime=-1
  Detect Increase1 : simulink/Logic and Bit Operations/Detect Increase  vinit=0  OutDataTypeStr=boolean
      settings: LibrarySourceBlock=|
      | hdlsllib/Logic and Bit
      | Operations/Detect
      | Increase
  Display : Display
  HDL Counter : hdlsllib/Sources/HDL Counter  CountType=Count limited  CountInit=0  CountStep=1  CountMax=65535  CountFromType=Initial value  CountFrom=0  CountResetPort=on  CountLoadPort=off  CountEnbPort=on  CountDirPort=off  CountHitOutputPort=off  CountDataType=Unsigned  CountWordLen=16  CountFracLen=0  CountSampTime=1
  Logical Operator1 : Logic  Operator=NOT  AllPortsSameDT=off  OutDataTypeStr=boolean
  Switch : Switch  Criteria=u2 ~= 0  SaturateOnIntegerOverflow=off  InputSameDT=off
  nsproduct : Product  OutDataTypeStr=uint32  RndMeth=Simplest
  posage : Outport  OutDataTypeStr=uint32
  wires:
  wrok/1 -> Switch/3
  Detect Increase1/1 -> HDL Counter/1, Logical Operator1/1
  Constant/1 -> nsproduct/1
  nsproduct/1 -> posage/1  "ns elapsed"
  Logical Operator1/1 -> HDL Counter/2
  HDL Counter/1 -> Display/1, nsproduct/2
  recieving/1 -> Switch/1
  Switch/1 -> Detect Increase1/1
  altmode/1 -> Switch/2

== system UZ_EnDat_be4_adding_bidirectional_clk_shift/UZ_ENDAT/ramselektor ==
  In1 : Inport  OutMin=0  OutMax=15  OutDataTypeStr=fixdt(0,4,0, 'DataTypeOverride', 'Off')  LockScale=on
  Trigger : TriggerPort  VariantControl=(inherit)  OutputDataType=int8  InitialTriggerSignalState=positive
  Delay : Delay  DelayLength=99
  Increment Stored Integer : hdlsllib/Math Operations/Increment Stored Integer
  SEL : Outport  InitialOutput=0
  wires:
  In1/1 -> Delay/1
  Increment Stored Integer/1 -> SEL/1
  Delay/1 -> Increment Stored Integer/1

== system UZ_EnDat_be4_adding_bidirectional_clk_shift/UZ_ENDAT/signalquality ==
  wrok : Inport  OutDataTypeStr=boolean
  payload : Inport  Port=2
  dbg2 : Inport  Port=3
  Bit Slice1 : hdlsllib/Logic and Bit Operations/Bit Slice  lidx=0  ridx=0
  Compare To Constant1 : hdlsllib/Logic and Bit Operations/Compare To Constant  relop=>  const=15  OutDataTypeStr=boolean
  Compare To Constant2 : hdlsllib/Logic and Bit Operations/Compare To Constant  relop=<  const=37  OutDataTypeStr=boolean
  Compare To Zero : hdlsllib/Logic and Bit Operations/Compare To Zero  relop=>  OutDataTypeStr=boolean
  Data Type Conversion1 : DataTypeConversion  OutDataTypeStr=boolean  SaturateOnIntegerOverflow=off  RndMeth=Floor
  Data Type Conversion4 : DataTypeConversion  OutDataTypeStr=uint32  RndMeth=Simplest  SaturateOnIntegerOverflow=off
  Delay : Delay  DelayLength=1
  Detect Increase1 : simulink/Logic and Bit Operations/Detect Increase  vinit=0  OutDataTypeStr=boolean
      settings: LibrarySourceBlock=|
      | hdlsllib/Logic and Bit
      | Operations/Detect
      | Increase
  Display : Display
      settings: Format=hex (Stored Integer)
  Display1 : Display
      settings: Format=hex (Stored Integer)
  HDL Counter : hdlsllib/Sources/HDL Counter  CountType=Count limited  CountInit=0  CountStep=1  CountMax=100000000  CountFromType=Initial value  CountFrom=0  CountResetPort=off  CountLoadPort=off  CountEnbPort=off  CountDirPort=off  CountHitOutputPort=on  CountDataType=Unsigned  CountWordLen=32  CountFracLen=0  CountSampTime=-1
  HDL Counter1 : hdlsllib/Sources/HDL Counter  CountType=Free running  CountInit=0  CountStep=1  CountMax=10000000  CountFromType=Initial value  CountFrom=0  CountResetPort=on  CountLoadPort=off  CountEnbPort=on  CountDirPort=off  CountHitOutputPort=off  CountDataType=Unsigned  CountWordLen=16  CountFracLen=0  CountSampTime=-1
  Logical Operator8 : Logic  Inputs=5  AllPortsSameDT=off  OutDataTypeStr=boolean
  Switch1 : Switch  Criteria=u2 ~= 0  SaturateOnIntegerOverflow=off  InputSameDT=off
  Terminator : Terminator
  amoundofsyncs : Outport  OutDataTypeStr=uint16
  wires:
  Detect Increase1/1 -> HDL Counter1/2
  HDL Counter/1 -> Terminator/1
  wrok/1 -> Logical Operator8/1
  HDL Counter/2 -> Switch1/2, HDL Counter1/1
  HDL Counter1/1 -> Switch1/1
  Switch1/1 -> Delay/1, amoundofsyncs/1
  Delay/1 -> Switch1/3
  Logical Operator8/1 -> Detect Increase1/1
  Compare To Zero/1 -> Logical Operator8/2
  dbg2/1 -> Compare To Constant1/1, Compare To Constant2/1
  Compare To Constant1/1 -> Logical Operator8/3
  Compare To Constant2/1 -> Logical Operator8/5
  payload/1 -> Display/1, Data Type Conversion4/1, Bit Slice1/1
  Data Type Conversion4/1 -> Display1/1, Compare To Zero/1
  Bit Slice1/1 -> Data Type Conversion1/1
  Data Type Conversion1/1 -> Logical Operator8/4

== system UZ_EnDat_be4_adding_bidirectional_clk_shift/UZ_ENDAT/timingprovider ==
  wrok : Inport  OutDataTypeStr=boolean
  clk : Inport  Port=2  OutDataTypeStr=boolean
  Compare To Constant1 : hdlsllib/Logic and Bit Operations/Compare To Constant  relop===  const=0  OutDataTypeStr=boolean
  Constant3 : Constant  Commented=on  Value=0x7FFFF0  OutDataTypeStr=uint32  SampleTime=-1
  Constant4 : Constant  Commented=on  Value=0x7FFFFF  OutDataTypeStr=uint32  SampleTime=-1
  Logical Operator : Logic  Operator=OR  AllPortsSameDT=off  OutDataTypeStr=boolean
  Subsystem1 : Subsystem
  Subsystem2 : Subsystem  Commented=on
  Subsystem3 : Subsystem
  Subsystem4 : Subsystem
  Subsystem5 : Subsystem  Commented=on
  Subsystem6 : Subsystem  Commented=on
  Subsystem7 : Subsystem
  timeelapsed2cycl : Outport  OutDataTypeStr=uint32
  timeelapsed1cycl : Outport  Port=2  OutDataTypeStr=uint32
  wires:
  wrok/1 -> Subsystem1/Trigger
  Subsystem3/1(ns elapsed) -> timeelapsed2cycl/1
  Subsystem7/1(ns elapsed) -> timeelapsed1cycl/1
  Subsystem1/1(valin1) -> Compare To Constant1/1, Subsystem7/1(elapsed), Subsystem3/1(elapsed)
  Logical Operator/1 -> Subsystem4/1(reset)
  Compare To Constant1/1 -> Logical Operator/2
  clk/1 -> Subsystem4/Trigger
  Subsystem4/1(valin1) -> Subsystem7/2(clkcnt), Subsystem3/2(clkcnt)
  Subsystem1/2(valin2) -> Logical Operator/1

== system UZ_EnDat_be4_adding_bidirectional_clk_shift/UZ_ENDAT/timingprovideralternative ==
  wrok : Inport  OutDataTypeStr=boolean
  clk : Inport  Port=2  OutDataTypeStr=boolean
  Compare To Constant1 : hdlsllib/Logic and Bit Operations/Compare To Constant  relop===  const=0  OutDataTypeStr=boolean
  Constant3 : Constant  Commented=on  Value=0x7FFFF0  OutDataTypeStr=uint32  SampleTime=-1
  Constant4 : Constant  Commented=on  Value=0x7FFFFF  OutDataTypeStr=uint32  SampleTime=-1
  Logical Operator : Logic  Operator=OR  AllPortsSameDT=off  OutDataTypeStr=boolean
  Subsystem1 : Subsystem
  Subsystem2 : Subsystem
  Subsystem3 : Subsystem
  Subsystem4 : Subsystem
  Terminator : Terminator
  timingproviderold : Subsystem  Commented=on
      settings: LibrarySourceBlock=|
      | hdlsllib/Ports &
      | Subsystems/Subsystem
  timeelapsed2cycl : Outport  OutDataTypeStr=uint32
  timeelapsed1cycl : Outport  Port=2  OutDataTypeStr=uint32
  wires:
  wrok/1 -> Subsystem1/Trigger
  Subsystem2/1(ns elapsed) -> timeelapsed2cycl/1
  Subsystem3/1(ns elapsed) -> timeelapsed1cycl/1
  Subsystem1/1(valin1) -> Compare To Constant1/1, Subsystem3/1(elapsed), Subsystem2/1(elapsed)
  Logical Operator/1 -> Subsystem4/1(reset)
  Compare To Constant1/1 -> Logical Operator/2
  clk/1 -> Terminator/1
  Subsystem4/1(valin1) -> Subsystem2/2(clkcnt), Subsystem3/2(clkcnt)
  Subsystem1/2(valin2) -> Logical Operator/1

== system UZ_EnDat_be4_adding_bidirectional_clk_shift/UZ_ENDAT/timingproviderold1 ==
  wrok : Inport  OutDataTypeStr=boolean
  clk : Inport  Port=2  OutDataTypeStr=boolean
  Compare To Constant1 : hdlsllib/Logic and Bit Operations/Compare To Constant  relop===  const=0  OutDataTypeStr=boolean
  Constant3 : Constant  Commented=on  Value=0x7FFFF0  OutDataTypeStr=uint32  SampleTime=-1
  Constant4 : Constant  Commented=on  Value=0x7FFFFF  OutDataTypeStr=uint32  SampleTime=-1
  Logical Operator : Logic  Operator=OR  AllPortsSameDT=off  OutDataTypeStr=boolean
  Subsystem1 : Subsystem
  Subsystem2 : Subsystem
  Subsystem3 : Subsystem
  Subsystem4 : Subsystem
  timeelapsed2cycl : Outport  OutDataTypeStr=uint32
  timeelapsed1cycl : Outport  Port=2  OutDataTypeStr=uint32
  wires:
  wrok/1 -> Subsystem1/Trigger
  Subsystem2/1(ns elapsed) -> timeelapsed2cycl/1
  Subsystem3/1(ns elapsed) -> timeelapsed1cycl/1
  Subsystem1/1(valin1) -> Compare To Constant1/1, Subsystem3/1(elapsed), Subsystem2/1(elapsed)
  Logical Operator/1 -> Subsystem4/1(reset)
  Compare To Constant1/1 -> Logical Operator/2
  clk/1 -> Subsystem4/Trigger
  Subsystem4/1(valin1) -> Subsystem2/2(clkcnt), Subsystem3/2(clkcnt)
  Subsystem1/2(valin2) -> Logical Operator/1

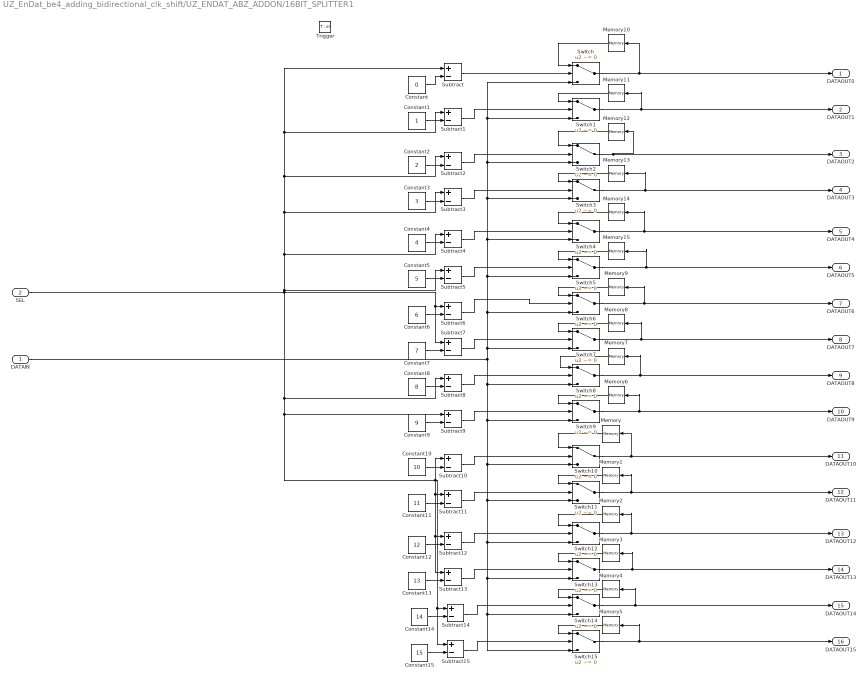
== system UZ_EnDat_be4_adding_bidirectional_clk_shift/UZ_ENDAT_ABZ_ADDON/16BIT_SPLITTER1 ==
  DATAIN : Inport
  SEL : Inport  Port=2  OutDataTypeStr=fixdt(0,4,0)
  Trigger : TriggerPort  TriggerType=falling  VariantControl=(inherit)  OutputDataType=int8  InitialTriggerSignalState=positive
  Constant : Constant  Value=0  OutDataTypeStr=fixdt(0,4,0)  SampleTime=-1
  Constant1 : Constant  OutDataTypeStr=fixdt(0,4,0)  SampleTime=-1
  Constant10 : Constant  Value=10  OutDataTypeStr=fixdt(0,4,0)  SampleTime=-1
  Constant11 : Constant  Value=11  OutDataTypeStr=fixdt(0,4,0)  SampleTime=-1
  Constant12 : Constant  Value=12  OutDataTypeStr=fixdt(0,4,0)  SampleTime=-1
  Constant13 : Constant  Value=13  OutDataTypeStr=fixdt(0,4,0)  SampleTime=-1
  Constant14 : Constant  Value=14  OutDataTypeStr=fixdt(0,4,0)  SampleTime=-1
  Constant15 : Constant  Value=15  OutDataTypeStr=fixdt(0,4,0)  SampleTime=-1
  Constant2 : Constant  Value=2  OutDataTypeStr=fixdt(0,4,0)  SampleTime=-1
  Constant3 : Constant  Value=3  OutDataTypeStr=fixdt(0,4,0)  SampleTime=-1
  Constant4 : Constant  Value=4  OutDataTypeStr=fixdt(0,4,0)  SampleTime=-1
  Constant5 : Constant  Value=5  OutDataTypeStr=fixdt(0,4,0)  SampleTime=-1
  Constant6 : Constant  Value=6  OutDataTypeStr=fixdt(0,4,0)  SampleTime=-1
  Constant7 : Constant  Value=7  OutDataTypeStr=fixdt(0,4,0)  SampleTime=-1
  Constant8 : Constant  Value=8  OutDataTypeStr=fixdt(0,4,0)  SampleTime=-1
  Constant9 : Constant  Value=9  OutDataTypeStr=fixdt(0,4,0)  SampleTime=-1
  Memory{,1..8,10..11} (11 alike) : Memory  InheritSampleTime=on
  Memory{9,12..15} (5 alike) : Memory  InitialCondition=100  InheritSampleTime=on  LinearizeAsDelay=on
  Subtract{,1..9,11..15} (15 alike) : Sum  Inputs=+-  OutDataTypeStr=fixdt(0,4,0)
  Subtract10 : Sum  Inputs=+-  AccumDataTypeStr=fixdt(0,4,0)
  Switch{,1..15} (16 alike) : Switch  Criteria=u2 ~= 0  SaturateOnIntegerOverflow=off  InputSameDT=off
  DATAOUT0 : Outport  InitialOutput=0
  DATAOUT1 : Outport  Port=2  InitialOutput=0
  DATAOUT2 : Outport  Port=3  InitialOutput=0
  DATAOUT3 : Outport  Port=4  InitialOutput=0
  DATAOUT4 : Outport  Port=5  InitialOutput=0
  DATAOUT5 : Outport  Port=6  InitialOutput=0
  DATAOUT6 : Outport  Port=7  InitialOutput=0
  DATAOUT7 : Outport  Port=8  InitialOutput=0
  DATAOUT8 : Outport  Port=9  InitialOutput=0
  DATAOUT9 : Outport  Port=10  InitialOutput=0
  DATAOUT10 : Outport  Port=11  InitialOutput=0
  DATAOUT11 : Outport  Port=12  InitialOutput=0
  DATAOUT12 : Outport  Port=13  InitialOutput=0
  DATAOUT13 : Outport  Port=14  InitialOutput=0
  DATAOUT14 : Outport  Port=15  InitialOutput=0
  DATAOUT15 : Outport  Port=16  InitialOutput=0
  wires:
  Switch/1 -> Memory10/1, DATAOUT0/1
  Switch1/1 -> Memory11/1, DATAOUT1/1
  Switch3/1 -> Memory13/1, DATAOUT3/1
  Switch2/1 -> Memory12/1, DATAOUT2/1
  Switch5/1 -> Memory15/1, DATAOUT5/1
  Switch4/1 -> Memory14/1, DATAOUT4/1
  Switch7/1 -> Memory8/1, DATAOUT7/1
  Switch6/1 -> Memory9/1, DATAOUT6/1
  Switch9/1 -> Memory6/1, DATAOUT9/1
  Switch10/1 -> Memory/1, DATAOUT10/1
  Switch11/1 -> Memory1/1, DATAOUT11/1
  Switch8/1 -> Memory7/1, DATAOUT8/1
  Switch12/1 -> Memory2/1, DATAOUT12/1
  Switch15/1 -> Memory5/1, DATAOUT15/1
  Switch13/1 -> Memory3/1, DATAOUT13/1
  Switch14/1 -> Memory4/1, DATAOUT14/1
  Constant/1 -> Subtract/2
  Subtract/1 -> Switch/2
  Subtract1/1 -> Switch1/2
  Constant1/1 -> Subtract1/2
  Constant2/1 -> Subtract2/2
  Subtract2/1 -> Switch2/2
  Constant3/1 -> Subtract3/2
  Subtract3/1 -> Switch3/2
  Constant4/1 -> Subtract4/2
  Subtract4/1 -> Switch4/2
  Constant5/1 -> Subtract5/2
  Subtract5/1 -> Switch5/2
  Constant6/1 -> Subtract6/2
  Subtract6/1 -> Switch6/2
  Constant7/1 -> Subtract7/2
  Subtract7/1 -> Switch7/2
  Constant8/1 -> Subtract8/2
  Subtract8/1 -> Switch8/2
  Constant9/1 -> Subtract9/2
  Subtract9/1 -> Switch9/2
  Constant10/1 -> Subtract10/2
  Subtract10/1 -> Switch10/2
  Constant11/1 -> Subtract11/2
  Subtract11/1 -> Switch11/2
  Constant12/1 -> Subtract12/2
  Subtract12/1 -> Switch12/2
  Constant13/1 -> Subtract13/2
  Subtract13/1 -> Switch13/2
  Constant14/1 -> Subtract14/2
  Subtract14/1 -> Switch14/2
  Constant15/1 -> Subtract15/2
  SEL/1 -> Subtract15/1, Subtract14/1, Subtract13/1, Subtract12/1, Subtract11/1, Subtract10/1, Subtract9/1, Subtract8/1, Subtract7/1, Subtract6/1, Subtract5/1, Subtract4/1, Subtract3/1, Subtract2/1, Subtract1/1, Subtract/1
  Subtract15/1 -> Switch15/2
  DATAIN/1 -> Switch4/3, Switch3/3, Switch2/3, Switch1/3, Switch/3, Switch5/3, Switch6/3, Switch7/3, Switch9/3, Switch10/3, Switch11/3, Switch12/3, Switch14/3, Switch15/3, Switch13/3, Switch8/3
  Memory/1 -> Switch10/1
  Memory1/1 -> Switch11/1
  Memory2/1 -> Switch12/1
  Memory3/1 -> Switch13/1
  Memory4/1 -> Switch14/1
  Memory5/1 -> Switch15/1
  Memory6/1 -> Switch9/1
  Memory7/1 -> Switch8/1
  Memory8/1 -> Switch7/1
  Memory9/1 -> Switch6/1
  Memory10/1 -> Switch/1
  Memory11/1 -> Switch1/1
  Memory12/1 -> Switch2/1
  Memory13/1 -> Switch3/1
  Memory14/1 -> Switch4/1
  Memory15/1 -> Switch5/1

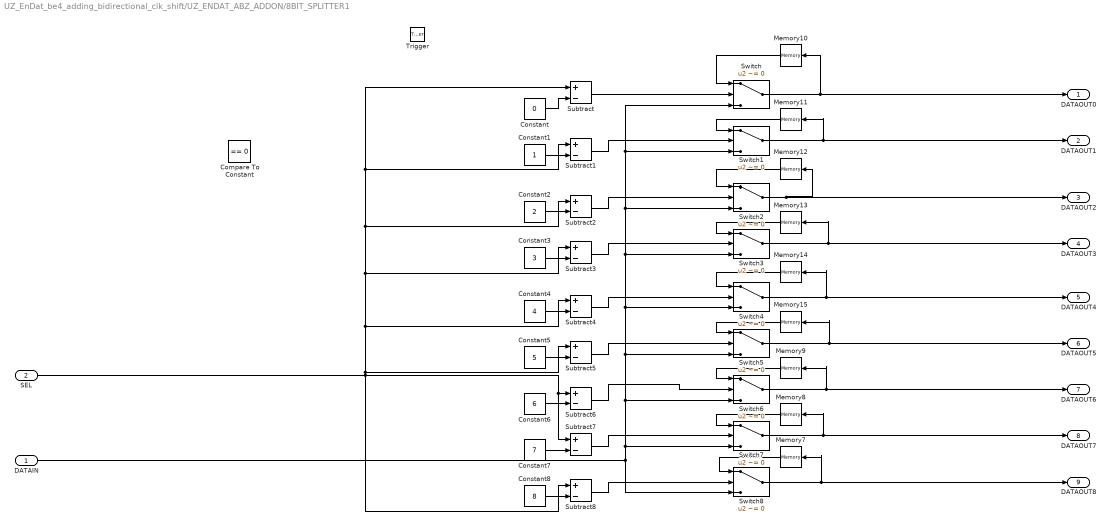
== system UZ_EnDat_be4_adding_bidirectional_clk_shift/UZ_ENDAT_ABZ_ADDON/8BIT_SPLITTER1 ==
  DATAIN : Inport
  SEL : Inport  Port=2  OutDataTypeStr=fixdt(0,4,0)
  Trigger : TriggerPort  TriggerType=falling  VariantControl=(inherit)  OutputDataType=int8  InitialTriggerSignalState=positive
  Compare To Constant : hdlsllib/Logic and Bit Operations/Compare To Constant  relop===  const=0  OutDataTypeStr=boolean
  Constant : Constant  Value=0  OutDataTypeStr=fixdt(0,4,0)  SampleTime=-1
  Constant1 : Constant  OutDataTypeStr=fixdt(0,4,0)  SampleTime=-1
  Constant2 : Constant  Value=2  OutDataTypeStr=fixdt(0,4,0)  SampleTime=-1
  Constant3 : Constant  Value=3  OutDataTypeStr=fixdt(0,4,0)  SampleTime=-1
  Constant4 : Constant  Value=4  OutDataTypeStr=fixdt(0,4,0)  SampleTime=-1
  Constant5 : Constant  Value=5  OutDataTypeStr=fixdt(0,4,0)  SampleTime=-1
  Constant6 : Constant  Value=6  OutDataTypeStr=fixdt(0,4,0)  SampleTime=-1
  Constant7 : Constant  Value=7  OutDataTypeStr=fixdt(0,4,0)  SampleTime=-1
  Constant8 : Constant  Value=8  OutDataTypeStr=fixdt(0,4,0)  SampleTime=-1
  Memory{7..8,10..11} (4 alike) : Memory  InheritSampleTime=on
  Memory{9,12..15} (5 alike) : Memory  InitialCondition=100  InheritSampleTime=on  LinearizeAsDelay=on
  Subtract{,1..8} (9 alike) : Sum  Inputs=+-  OutDataTypeStr=fixdt(0,4,0)
  Switch{,1..8} (9 alike) : Switch  Criteria=u2 ~= 0  SaturateOnIntegerOverflow=off  InputSameDT=off
  DATAOUT0 : Outport  InitialOutput=0
  DATAOUT1 : Outport  Port=2  InitialOutput=0
  DATAOUT2 : Outport  Port=3  InitialOutput=0
  DATAOUT3 : Outport  Port=4  InitialOutput=0
  DATAOUT4 : Outport  Port=5  InitialOutput=0
  DATAOUT5 : Outport  Port=6  InitialOutput=0
  DATAOUT6 : Outport  Port=7  InitialOutput=0
  DATAOUT7 : Outport  Port=8  InitialOutput=0
  DATAOUT8 : Outport  Port=9  InitialOutput=0
  wires:
  Switch/1 -> Memory10/1, DATAOUT0/1
  Switch1/1 -> Memory11/1, DATAOUT1/1
  Switch3/1 -> Memory13/1, DATAOUT3/1
  Switch2/1 -> Memory12/1, DATAOUT2/1
  Switch5/1 -> Memory15/1, DATAOUT5/1
  Switch4/1 -> Memory14/1, DATAOUT4/1
  Switch7/1 -> Memory8/1, DATAOUT7/1
  Switch6/1 -> Memory9/1, DATAOUT6/1
  Switch8/1 -> Memory7/1, DATAOUT8/1
  Constant/1 -> Subtract/2
  Subtract/1 -> Switch/2
  Subtract1/1 -> Switch1/2
  Constant1/1 -> Subtract1/2
  Constant2/1 -> Subtract2/2
  Subtract2/1 -> Switch2/2
  Constant3/1 -> Subtract3/2
  Subtract3/1 -> Switch3/2
  Constant4/1 -> Subtract4/2
  Subtract4/1 -> Switch4/2
  Constant5/1 -> Subtract5/2
  Subtract5/1 -> Switch5/2
  Constant6/1 -> Subtract6/2
  Subtract6/1 -> Switch6/2
  Constant7/1 -> Subtract7/2
  Subtract7/1 -> Switch7/2
  Constant8/1 -> Subtract8/2
  Subtract8/1 -> Switch8/2
  ? -> ?
  SEL/1 -> Subtract8/1, Subtract7/1, Subtract6/1, Subtract5/1, Subtract4/1, Subtract3/1, Subtract2/1, Subtract1/1, Subtract/1
  DATAIN/1 -> Switch4/3, Switch3/3, Switch2/3, Switch1/3, Switch/3, Switch5/3, Switch6/3, Switch7/3, Switch8/3
  Memory7/1 -> Switch8/1
  Memory8/1 -> Switch7/1
  Memory9/1 -> Switch6/1
  Memory10/1 -> Switch/1
  Memory11/1 -> Switch1/1
  Memory12/1 -> Switch2/1
  Memory13/1 -> Switch3/1
  Memory14/1 -> Switch4/1
  Memory15/1 -> Switch5/1

== system UZ_EnDat_be4_adding_bidirectional_clk_shift/UZ_ENDAT_ABZ_ADDON/DATA2CLOCKSYNCER1 ==
  In1 : Inport
  FAKTOR : Inport  Port=2
  Constant : Constant  Value=9999  OutDataTypeStr=uint16  SampleTime=-1
  Constant1 : Constant  Value=384  OutDataTypeStr=uint16  SampleTime=-1
  Constant2 : Constant  Value=5  OutDataTypeStr=uint16  SampleTime=-1
  Constant23 : Constant  Value=96  OutDataTypeStr=uint16  SampleTime=-1
  Constant24 : Constant  Value=192  OutDataTypeStr=uint16  SampleTime=-1
  Constant3 : Constant  Value=48  OutDataTypeStr=uint16  SampleTime=-1
  Constant4 : Constant  Value=11  OutDataTypeStr=uint16  SampleTime=-1
  Constant7 : Constant  Value=23  OutDataTypeStr=uint16  SampleTime=-1
  Display15 : Display
  Divide : Product  Inputs=*/  OutDataTypeStr=uint16  RndMeth=Simplest  SaturateOnIntegerOverflow=on  LockScale=on
  Multiport Switch1 : MultiPortSwitch  DataPortOrder=Zero-based contiguous  Inputs=7  DataPortIndices={8,16,32,64}  zeroidx=on  SaturateOnIntegerOverflow=off  InputSameDT=off
  Product : Product  RndMeth=Simplest  SaturateOnIntegerOverflow=on  OutDataTypeStr=Inherit: Same as first input
  Out1 : Outport
  wires:
  In1/1 -> Multiport Switch1/1
  FAKTOR/1 -> Product/2
  Constant/1 -> Divide/2
  Multiport Switch1/1 -> Product/1
  Product/1 -> Divide/1
  Constant2/1 -> Multiport Switch1/2
  Constant4/1 -> Multiport Switch1/3
  Constant7/1 -> Multiport Switch1/4
  Constant3/1 -> Multiport Switch1/5
  Constant23/1 -> Multiport Switch1/6
  Constant24/1 -> Multiport Switch1/7
  Constant1/1 -> Multiport Switch1/8
  Divide/1 -> Display15/1, Out1/1
